simulink model "task_simulation_wo_atan"  (R2025b)
settings: Solver=VariableStepDiscrete  StartTime=0.0  StopTime=10  FixedStep=0.001  MaxStep=0.0001  RelTol=1e-3
InitFcn:
  | prepare_parameters
undefined symbols (not defined in the file): DiscIntNeverNeededParam, I_max_val, J_1_val, J_2_val, k_E_val, k_M_val, k_t_val, L_val, R_val, U_max_val
libraries: slpidlib x2, embmathops x1, simulink_extras x1
settings Model: Creator=10120  LastModifiedBy=10120

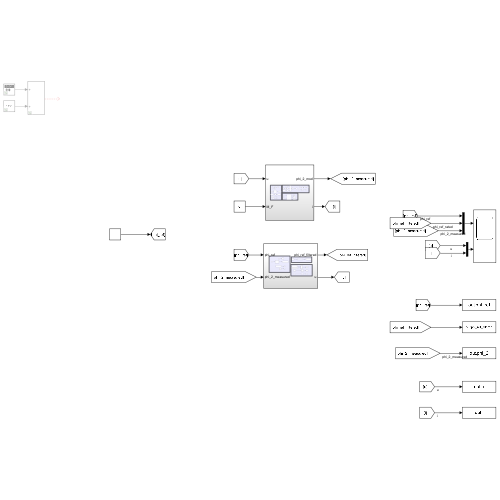
[thumbnail: Simulink's stored preview of the top-level diagram]
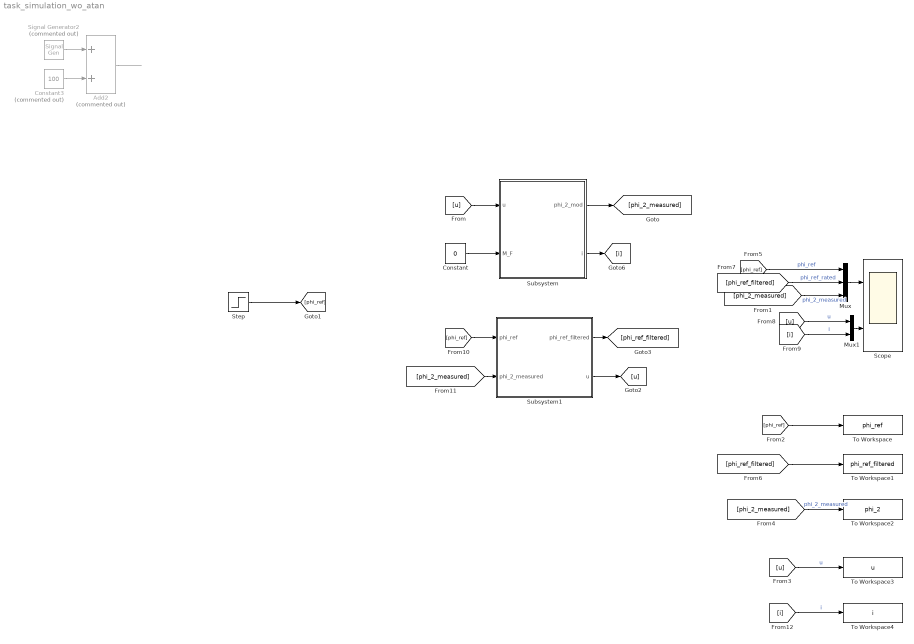
== system task_simulation_wo_atan ==
  Add2 : Sum  Commented=on
  Constant : Constant  Value=0
  Constant3 : Constant  Commented=on  Value=100
  Mux : Mux  Inputs=3
  Mux1 : Mux  Inputs=2
  Scope : Scope  NumInputPorts=2
      settings: ActiveDisplayYMinimum=-44.99891482188324  ActiveDisplayYMaximum=404.99023339694924
  Signal Generator2 : SignalGenerator  Commented=on  Amplitude=100  Frequency=0.1  Units=rad/sec
  Step : Step  Time=0.1  After=200  SampleTime=1e-4  mask(DiscretizedSource){}
      mask init:
      | %zoh
  Subsystem : Subsystem
  Subsystem1 : Subsystem
  To Workspace : ToWorkspace  VariableName=phi_ref  SaveFormat=Structure With Time  SampleTime=-1
  To Workspace1 : ToWorkspace  VariableName=phi_ref_filtered  SaveFormat=Structure With Time  SampleTime=-1
  To Workspace2 : ToWorkspace  VariableName=phi_2  SaveFormat=Structure With Time  SampleTime=-1
  To Workspace3 : ToWorkspace  VariableName=u  SaveFormat=Structure With Time  SampleTime=-1
  To Workspace4 : ToWorkspace  VariableName=i  SaveFormat=Structure With Time  SampleTime=-1
  wires:
  Constant/1 -> Subsystem/2(M_F)
  [u] -> Subsystem/1(u)
  Subsystem/1(phi_2_mod) -> [phi_2_measured]
  Step/1 -> [phi_ref]
  Add2/1 -> ?
  Constant3/1 -> Add2/2
  Signal Generator2/1 -> Add2/1
  Mux/1 -> Scope/1
  [phi_ref] -> Mux/1  "phi_ref"
  [phi_ref_filtered] -> Mux/2  "phi_ref_rated"
  [phi_2_measured] -> Mux/3  "phi_2_measured"
  Subsystem/2(i) -> [i]
  [phi_ref] -> Subsystem1/1(phi_ref)
  [phi_2_measured] -> Subsystem1/2(phi_2_measured)
  Subsystem1/2(u) -> [u]
  Subsystem1/1(phi_ref_filtered) -> [phi_ref_filtered]
  Mux1/1 -> Scope/2
  [u] -> Mux1/1  "u"
  [i] -> Mux1/2  "i"
  [phi_ref] -> To Workspace/1
  [phi_ref_filtered] -> To Workspace1/1
  [phi_2_measured] -> To Workspace2/1  "phi_2_measured"
  [u] -> To Workspace3/1  "u"
  [i] -> To Workspace4/1  "i"

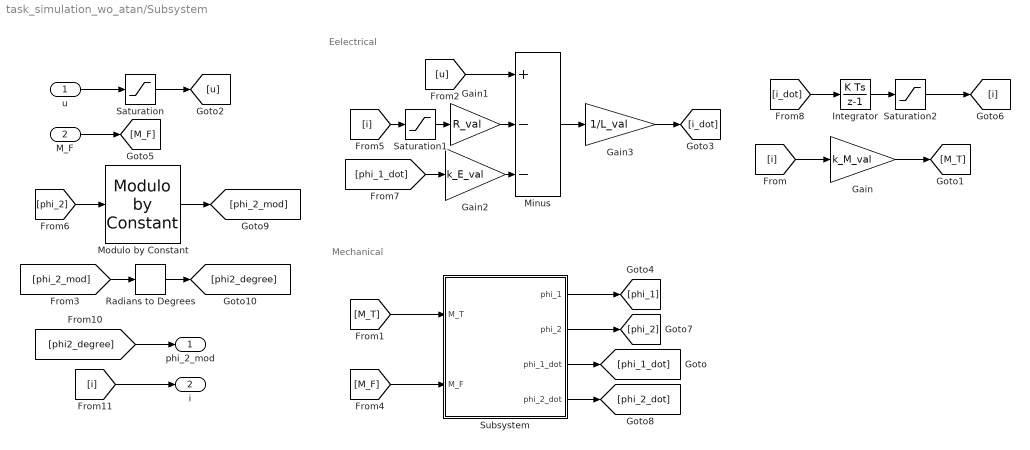
== system task_simulation_wo_atan/Subsystem ==
  note: Mechanical
  note: Eelectrical
  u : Inport
  M_F : Inport  Port=2
  Gain : Gain  Gain=k_M_val
  Gain1 : Gain  Gain=R_val
  Gain2 : Gain  Gain=k_E_val
  Gain3 : Gain  Gain=1/L_val
  Integrator : DiscreteIntegrator  SampleTime=1e-4  ICPrevOutput=DiscIntNeverNeededParam  ICPrevScaledInput=DiscIntNeverNeededParam  mask(DiscretizedDiscreteIntegrator){}
      mask init:
      | %zoh
  Minus : Sum  Inputs=+--
  Modulo by Constant : embmathops/Modulo by Constant  Denominator=2*pi  SimulateUsing=Code generation
      settings: LibrarySourceBlock=embeddedMathLib/Modulo by Constant
  Radians to Degrees : simulink_extras/Transformations/Radians to Degrees
  Saturation : Saturate  UpperLimit=U_max_val  LowerLimit=-U_max_val
  Saturation1 : Saturate  UpperLimit=I_max_val  LowerLimit=-I_max_val
  Saturation2 : Saturate  UpperLimit=I_max_val  LowerLimit=-I_max_val
  Subsystem : Subsystem
  phi_2_mod : Outport
  i : Outport  Port=2
  wires:
  [i] -> Gain/1
  Gain/1 -> [M_T]
  [M_T] -> Subsystem/1(M_T)
  u/1 -> Saturation/1
  Gain3/1 -> [i_dot]
  [u] -> Minus/1
  Gain1/1 -> Minus/2
  [i] -> Saturation1/1
  Subsystem/1(phi_1) -> [phi_1]
  Gain2/1 -> Minus/3
  [phi_1_dot] -> Gain2/1
  Minus/1 -> Gain3/1
  [i_dot] -> Integrator/1
  Integrator/1 -> Saturation2/1
  Subsystem/3(phi_1_dot) -> [phi_1_dot]
  [phi2_degree] -> phi_2_mod/1
  M_F/1 -> [M_F]
  [M_F] -> Subsystem/2(M_F)
  Subsystem/2(phi_2) -> [phi_2]
  Subsystem/4(phi_2_dot) -> [phi_2_dot]
  [phi_2] -> Modulo by Constant/1
  Modulo by Constant/1 -> [phi_2_mod]
  Saturation/1 -> [u]
  Saturation1/1 -> Gain1/1
  Saturation2/1 -> [i]
  [i] -> i/1
  [phi_2_mod] -> Radians to Degrees/1
  Radians to Degrees/1 -> [phi2_degree]

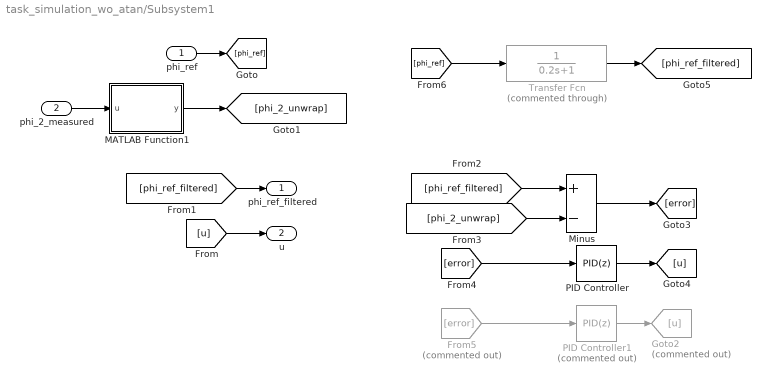
== system task_simulation_wo_atan/Subsystem1 ==
  phi_ref : Inport
  phi_2_measured : Inport  Port=2
  From5 : From  Commented=on  GotoTag=error
  Goto2 : Goto  Commented=on  GotoTag=u
  MATLAB Function1 : MATLAB Function  TreatAsAtomicUnit=on
  Minus : Sum  Inputs=+-
  PID Controller : slpidlib/PID Controller  Controller=PID  Form=Parallel  TimeDomain=Discrete-time  UseExternalTs=off  SampleTime=0.000100000000000000005  IntegratorMethod=Forward Euler  FilterMethod=Forward Euler  ControllerParametersSource=internal  P=0.020000000000000  I=0.000000000000000  UseKiTs=off  D=0.001388958334491  UseExternalDerivativeSource=off  N=0.999950001666638  UseFilter=off  TunerSelectOption=Transfer Function Based (PID Tuner App)  InitialConditionSource=internal  InitialConditionForIntegrator=0  InitialConditionForFilter=0  DifferentiatorICPrevScaledInput=0  ExternalReset=none  TrackingMode=off  Kt=1  LimitOutput=on  SatLimitsSource=internal  UpperSaturationLimit=U_max_val  LowerSaturationLimit=-U_max_val  LinearizeAsGain=on  AntiWindupMode=clamping  Kb=1  LimitIntegrator=off  UpperIntegratorSaturationLimit=inf  LowerIntegratorSaturationLimit=-inf  POutMin=[]  POutMax=[]  IOutMin=[]  IOutMax=[]  DOutMin=[]  DOutMax=[]  NOutMin=[]  NOutMax=[]  SumOutMin=[]  SumOutMax=[]  SaturationOutMin=[]  SaturationOutMax=[]  PParamMin=[]  PParamMax=[]  IParamMin=[]  IParamMax=[]  DParamMin=[]  DParamMax=[]  NParamMin=[]  NParamMax=[]  KbParamMin=[]  KbParamMax=[]  KtParamMin=[]  KtParamMax=[]  KbOutMin=[]  KbOutMax=[]  KtOutMin=[]  KtOutMax=[]  IntegratorOutMin=[]  IntegratorOutMax=[]  FilterOutMin=[]  FilterOutMax=[]  SumI1OutMin=[]  SumI1OutMax=[]  SumI2OutMin=[]  SumI2OutMax=[]  SumI3OutMin=[]  SumI3OutMax=[]  SumI4OutMin=[]  SumI4OutMax=[]  SumDOutMin=[]  SumDOutMax=[]  DifferentiatorOutMin=[]  DifferentiatorOutMax=[]  FilterDiffOutCoefMin=[]  FilterDiffOutCoefMax=[]  ReciprocalOutMin=[]  ReciprocalOutMax=[]  SumDenOutMin=[]  SumDenOutMax=[]  SumNumOutMin=[]  SumNumOutMax=[]  DivideOutMin=[]  DivideOutMax=[]  UdiffTsProdOutMin=[]  UdiffTsProdOutMax=[]  NTsProdOutMin=[]  NTsProdOutMax=[]  UintegralTsProdOutMin=[]  UintegralTsProdOutMax=[]  UngainTsProdOutMin=[]  UngainTsProdOutMax=[]  ClampingZeroOutDataTypeStr=Inherit: Inherit via back propagation  ClampingZeroOutMin=[]  ClampingZeroOutMax=[]  FilterDenConstantOutDataTypeStr=Inherit: Inherit via back propagation  FilterDenConstantOutMin=[]  FilterDenConstantOutMax=[]  PCopyOutDataTypeStr=Inherit: Inherit via back propagation  PCopyOutMin=[]  PCopyOutMax=[]  NCopyOutDataTypeStr=Inherit: Inherit via back propagation  NCopyOutMin=[]  NCopyOutMax=[]  IntegratorContinuousStateAttributes=''  IntegratorStateMustResolveToSignalObject=off  IntegratorRTWStateStorageClass=Auto  FilterContinuousStateAttributes=''  FilterStateMustResolveToSignalObject=off  FilterRTWStateStorageClass=Auto  ParallelPVariant=InternalParameters  IdealPVariant=Disabled  IVariant=InternalParameters  DVariant=InternalParameters  IntegratorVariant=Discrete  SatVariant=Enabled  AWVariant=DiscClampingParallel  PCopyVariant=Disabled  TRVariant=Disabled  FdbkBlocksVariant=Forward  IdealPFdbkVariant=Disabled  SatFdbkVariant=Disabled  DerivativeFilterVariant=Differentiator  NVariant=Passthrough  NCopyVariant=Disabled_SignalSpec  FilterICVariant=InternalICsDifferentiator  IntegratorICVariant=InternalICs  ExternalResetVariant=Disabled  TRSumVariant=Passthrough  SumFdbkVariant=Disabled  SumVariant=Sum_PID  TsampFilterVariant=InternalTs  TsampNgainVariant=Passthrough  TsampIntegralVariant=Disabled_SignalSpec  ExternalSaturationOutDataTypeStr=Inherit: Same as second input  DerivativeSourceVariant=ErrorSignal  PreIntVariant=InternalPreInt
  PID Controller1 : slpidlib/PID Controller  Commented=on  Controller=PID  Form=Parallel  TimeDomain=Discrete-time  UseExternalTs=off  SampleTime=0.000100000000000000005  IntegratorMethod=Forward Euler  FilterMethod=Forward Euler  ControllerParametersSource=internal  P=0.01  I=0.000000000000000  UseKiTs=off  D=0.000000000000000  UseExternalDerivativeSource=off  N=0.999950001666638  UseFilter=on  TunerSelectOption=Transfer Function Based (PID Tuner App)  InitialConditionSource=internal  InitialConditionForIntegrator=0  InitialConditionForFilter=0  DifferentiatorICPrevScaledInput=0  ExternalReset=none  TrackingMode=off  Kt=1  LimitOutput=on  SatLimitsSource=internal  UpperSaturationLimit=U_max_val  LowerSaturationLimit=-U_max_val  LinearizeAsGain=on  AntiWindupMode=clamping  Kb=1  LimitIntegrator=off  UpperIntegratorSaturationLimit=inf  LowerIntegratorSaturationLimit=-inf  POutMin=[]  POutMax=[]  IOutMin=[]  IOutMax=[]  DOutMin=[]  DOutMax=[]  NOutMin=[]  NOutMax=[]  SumOutMin=[]  SumOutMax=[]  SaturationOutMin=[]  SaturationOutMax=[]  PParamMin=[]  PParamMax=[]  IParamMin=[]  IParamMax=[]  DParamMin=[]  DParamMax=[]  NParamMin=[]  NParamMax=[]  KbParamMin=[]  KbParamMax=[]  KtParamMin=[]  KtParamMax=[]  KbOutMin=[]  KbOutMax=[]  KtOutMin=[]  KtOutMax=[]  IntegratorOutMin=[]  IntegratorOutMax=[]  FilterOutMin=[]  FilterOutMax=[]  SumI1OutMin=[]  SumI1OutMax=[]  SumI2OutMin=[]  SumI2OutMax=[]  SumI3OutMin=[]  SumI3OutMax=[]  SumI4OutMin=[]  SumI4OutMax=[]  SumDOutMin=[]  SumDOutMax=[]  DifferentiatorOutMin=[]  DifferentiatorOutMax=[]  FilterDiffOutCoefMin=[]  FilterDiffOutCoefMax=[]  ReciprocalOutMin=[]  ReciprocalOutMax=[]  SumDenOutMin=[]  SumDenOutMax=[]  SumNumOutMin=[]  SumNumOutMax=[]  DivideOutMin=[]  DivideOutMax=[]  UdiffTsProdOutMin=[]  UdiffTsProdOutMax=[]  NTsProdOutMin=[]  NTsProdOutMax=[]  UintegralTsProdOutMin=[]  UintegralTsProdOutMax=[]  UngainTsProdOutMin=[]  UngainTsProdOutMax=[]  ClampingZeroOutDataTypeStr=Inherit: Inherit via back propagation  ClampingZeroOutMin=[]  ClampingZeroOutMax=[]  FilterDenConstantOutDataTypeStr=Inherit: Inherit via back propagation  FilterDenConstantOutMin=[]  FilterDenConstantOutMax=[]  PCopyOutDataTypeStr=Inherit: Inherit via back propagation  PCopyOutMin=[]  PCopyOutMax=[]  NCopyOutDataTypeStr=Inherit: Inherit via back propagation  NCopyOutMin=[]  NCopyOutMax=[]  IntegratorContinuousStateAttributes=''  IntegratorStateMustResolveToSignalObject=off  IntegratorRTWStateStorageClass=Auto  FilterContinuousStateAttributes=''  FilterStateMustResolveToSignalObject=off  FilterRTWStateStorageClass=Auto  ParallelPVariant=InternalParameters  IdealPVariant=Disabled  IVariant=InternalParameters  DVariant=InternalParameters  IntegratorVariant=Discrete  SatVariant=Enabled  AWVariant=DiscClampingParallel  PCopyVariant=Disabled  TRVariant=Disabled  FdbkBlocksVariant=Forward  IdealPFdbkVariant=Disabled  SatFdbkVariant=Disabled  DerivativeFilterVariant=ForwardEulerFilter  NVariant=InternalParameters  NCopyVariant=Disabled  FilterICVariant=InternalICsFilter  IntegratorICVariant=InternalICs  ExternalResetVariant=Disabled  TRSumVariant=Passthrough  SumFdbkVariant=Disabled  SumVariant=Sum_PID  TsampFilterVariant=InternalTs  TsampNgainVariant=Passthrough  TsampIntegralVariant=Disabled_SignalSpec  ExternalSaturationOutDataTypeStr=Inherit: Same as second input  DerivativeSourceVariant=ErrorSignal  PreIntVariant=InternalPreInt
  Transfer Fcn : TransferFcn  Commented=through  Denominator=[0.2 1]
  phi_ref_filtered : Outport
  u : Outport  Port=2
  wires:
  Minus/1 -> [error]
  PID Controller/1 -> [u]
  [error] -> PID Controller/1
  Transfer Fcn/1 -> [phi_ref_filtered]
  [phi_2_unwrap] -> Minus/2
  [phi_ref] -> Transfer Fcn/1
  [phi_ref_filtered] -> Minus/1
  phi_ref/1 -> [phi_ref]
  [phi_ref_filtered] -> phi_ref_filtered/1
  [u] -> u/1
  PID Controller1/1 -> Goto2/1
  From5/1 -> PID Controller1/1
  phi_2_measured/1 -> MATLAB Function1/1(u)
  MATLAB Function1/1(y) -> [phi_2_unwrap]

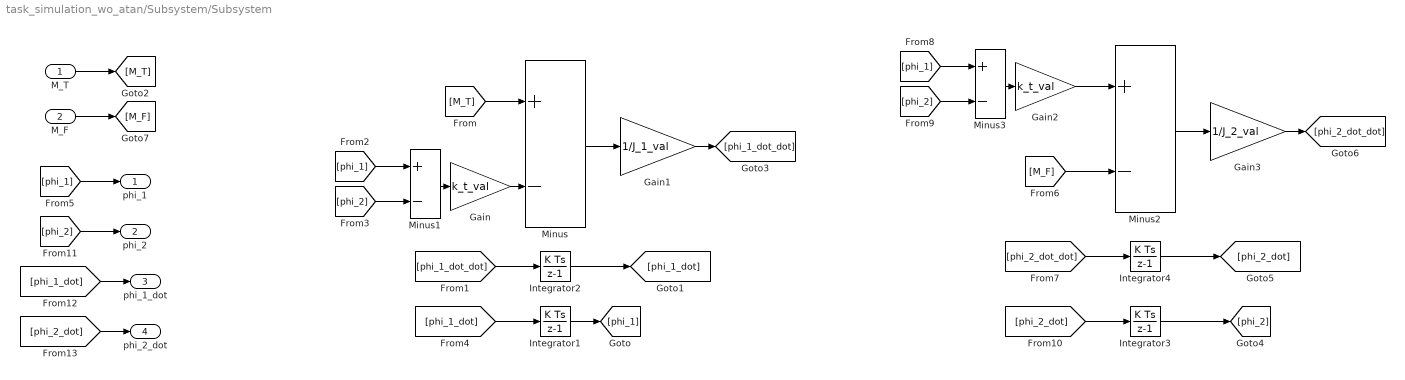
== system task_simulation_wo_atan/Subsystem/Subsystem ==
  M_T : Inport
  M_F : Inport  Port=2
  Gain : Gain  Gain=k_t_val
  Gain1 : Gain  Gain=1/J_1_val
  Gain2 : Gain  Gain=k_t_val
  Gain3 : Gain  Gain=1/J_2_val
  Integrator1 : DiscreteIntegrator  SampleTime=1e-4  ICPrevOutput=DiscIntNeverNeededParam  ICPrevScaledInput=DiscIntNeverNeededParam  mask(DiscretizedDiscreteIntegrator){}
      mask init:
      | %zoh
  Integrator2 : DiscreteIntegrator  SampleTime=1e-4  ICPrevOutput=DiscIntNeverNeededParam  ICPrevScaledInput=DiscIntNeverNeededParam  mask(DiscretizedDiscreteIntegrator){}
      mask init:
      | %zoh
  Integrator3 : DiscreteIntegrator  SampleTime=1e-4  ICPrevOutput=DiscIntNeverNeededParam  ICPrevScaledInput=DiscIntNeverNeededParam  mask(DiscretizedDiscreteIntegrator){}
      mask init:
      | %zoh
  Integrator4 : DiscreteIntegrator  SampleTime=1e-4  ICPrevOutput=DiscIntNeverNeededParam  ICPrevScaledInput=DiscIntNeverNeededParam  mask(DiscretizedDiscreteIntegrator){}
      mask init:
      | %zoh
  Minus{,1..3} (4 alike) : Sum  Inputs=+-
  phi_1 : Outport
  phi_2 : Outport  Port=2
  phi_1_dot : Outport  Port=3
  phi_2_dot : Outport  Port=4
  wires:
  [phi_1_dot] -> Integrator1/1
  Integrator1/1 -> [phi_1]
  Integrator2/1 -> [phi_1_dot]
  [phi_1_dot_dot] -> Integrator2/1
  M_T/1 -> [M_T]
  [M_T] -> Minus/1
  Minus1/1 -> Gain/1
  [phi_1] -> Minus1/1
  [phi_2] -> Minus1/2
  Gain/1 -> Minus/2
  Minus/1 -> Gain1/1
  Gain1/1 -> [phi_1_dot_dot]
  [phi_1] -> phi_1/1
  [phi_2_dot] -> Integrator3/1
  Integrator3/1 -> [phi_2]
  [phi_2_dot_dot] -> Integrator4/1
  Minus2/1 -> Gain3/1
  [phi_2] -> Minus3/2
  Integrator4/1 -> [phi_2_dot]
  Minus3/1 -> Gain2/1
  Gain3/1 -> [phi_2_dot_dot]
  [phi_1] -> Minus3/1
  Gain2/1 -> Minus2/1
  M_F/1 -> [M_F]
  [M_F] -> Minus2/2
  [phi_2] -> phi_2/1
  [phi_1_dot] -> phi_1_dot/1
  [phi_2_dot] -> phi_2_dot/1

== matlab function task_simulation_wo_atan/Subsystem1/MATLAB Function1 ==
  data: u input; y output
function y = unwrap_deg(u)
%#codegen
% Real-time unwrap for angle in degrees (0~360 input)
% Output: continuous angle in degrees

persistent prev_u prev_y initialized

if isempty(initialized)
    prev_u = u;
    prev_y = u;
    initialized = true;
    y = u;
    return
end

% 计算当前与上一次测量的差值
delta = u - prev_u;

% 将差值限制到 (-180, 180]
delta = mod(delta + 180, 360) - 180;

% 累加得到连续角度
y = prev_y + delta;

% 更新状态
prev_u = u;
prev_y = y;

end
